simulink model "itu801_luma_chroma_fir_12bit"  (Simulink 5.0)
settings: Solver=ode45  StartTime=0.0  StopTime=60  RelTol=1e-3
libraries: simulink x4
settings Model: LastModifiedBy=thh

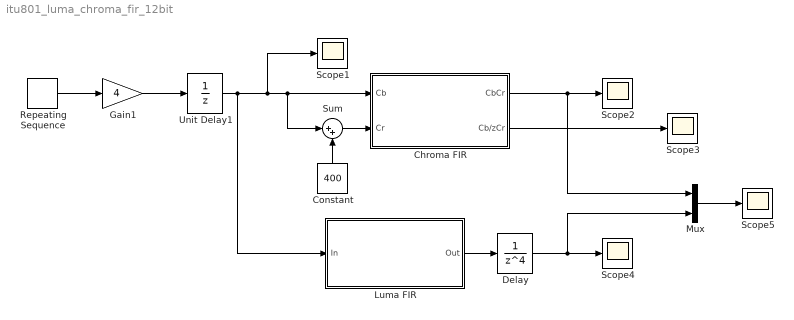
== system itu801_luma_chroma_fir_12bit ==
  Chroma FIR : Subsystem
  Constant : Constant  Orientation=up  Value=400
  Delay : DiscreteTransferFcn  Denominator=[1 0 0 0 0]
  Gain1 : Gain  Gain=4  SaturateOnIntegerOverflow=on
  Luma FIR : Subsystem
  Mux : Mux  Inputs=2
  Repeating Sequence : simulink/Sources/Repeating Sequence  rep_seq_t=[0 19 20 39 40]  rep_seq_y=[16 16 235 235 16]
  Scope{1..5} (5 alike) : Scope
      Scope1 settings: TimeRange=160  YMin=-0.2  YMax=1.2
      Scope2 settings: TimeRange=160  YMin=-1.5  YMax=4.5
      Scope3 settings: TimeRange=60  YMin=-0.2  YMax=1.2  SaveName=ScopeData3
      Scope4 settings: TimeRange=160  YMin=-0.2  YMax=1.2  SaveName=ScopeData2
      Scope5 settings: TimeRange=60  YMin=0  YMax=350  SaveName=ScopeData4
  Sum : Sum  Inputs=|++  SaturateOnIntegerOverflow=on
  Unit Delay1 : UnitDelay
  wires:
  Repeating Sequence/1 -> Gain1/1
  Sum/1 -> Chroma FIR/2(Cr)
  Constant/1 -> Sum/2
  Unit Delay1/1 -> Chroma FIR/1(Cb), Sum/1, Scope1/1, Luma FIR/1(In)
  Chroma FIR/2(Cb/zCr) -> Scope3/1
  Luma FIR/1(Out) -> Delay/1
  Mux/1 -> Scope5/1
  Gain1/1 -> Unit Delay1/1
  Delay/1 -> Scope4/1, Mux/2
  Chroma FIR/1(CbCr) -> Mux/1, Scope2/1

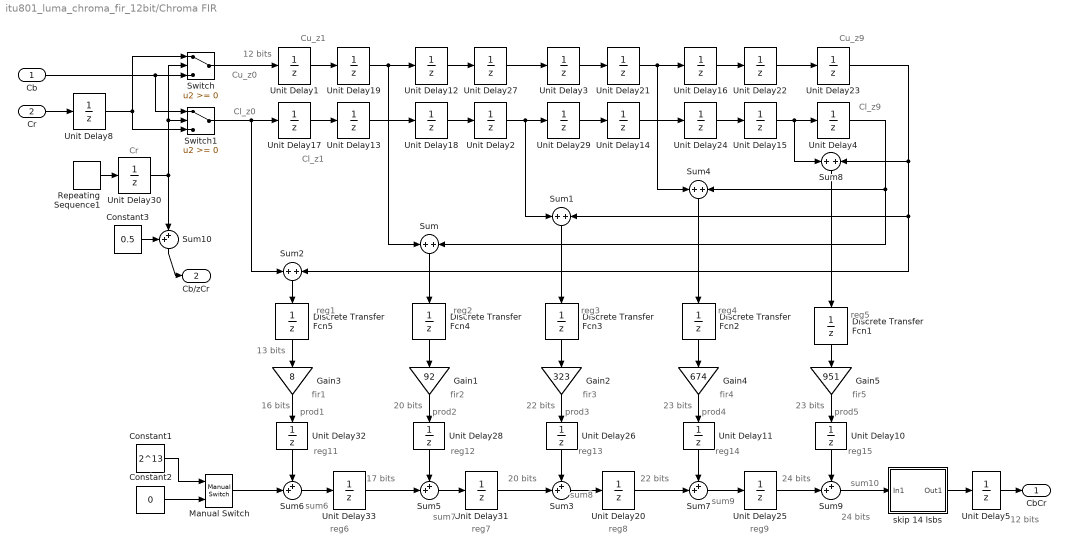
== system itu801_luma_chroma_fir_12bit/Chroma FIR ==
  note: fir1
  note: fir2
  note: fir3
  note: fir4
  note: fir5
  note: Cr
  note: 12 bits
  note: 13 bits
  note: Cu_z1
  note: Cu_z9
  note: Cl_z1
  note: Cl_z9
  note: 17 bits
  note: 20 bits
  note: 22 bits
  note: 24 bits
  note: 24 bits
  note: 12 bits
  note: reg1
  note: reg2
  note: reg3
  note: reg4
  note: reg5
  note: reg6
  note: reg7
  note: reg8
  note: reg9
  note: Cu_z0
  note: Cl_z0
  note: prod1
  note: prod2
  note: prod3
  note: prod4
  note: prod5
  note: reg11
  note: reg12
  note: reg13
  note: reg14
  note: reg15
  note: sum6
  note: sum7
  note: sum8
  note: sum9
  note: sum10
  note: 16 bits
  note: 20 bits
  note: 22 bits
  note: 23 bits
  note: 23 bits
  Cb : Inport
  Cr : Inport  Port=2
  Constant1 : Constant  Value=2^13
  Constant2 : Constant  Value=0
  Constant3 : Constant  Value=0.5
  Discrete Transfer Fcn{1..5} (5 alike) : DiscreteTransferFcn  Orientation=down  Denominator=[1 0]
  Gain1 : Gain  Orientation=down  Gain=92  SaturateOnIntegerOverflow=on
  Gain2 : Gain  Orientation=down  Gain=323  SaturateOnIntegerOverflow=on
  Gain3 : Gain  Orientation=down  Gain=8  SaturateOnIntegerOverflow=on
  Gain4 : Gain  Orientation=down  Gain=674  SaturateOnIntegerOverflow=on
  Gain5 : Gain  Orientation=down  Gain=951  SaturateOnIntegerOverflow=on
  Manual Switch : simulink/Signal Routing/Manual Switch  sw=1  action=0
  Repeating Sequence1 : simulink/Sources/Repeating Sequence  rep_seq_t=[0 1 2]  rep_seq_y=[0.5 -0.5 0.5]
  Sum{,1..2,4,8} (5 alike) : Sum  Orientation=down  SaturateOnIntegerOverflow=on
  Sum10 : Sum  Orientation=down  Inputs=++|  SaturateOnIntegerOverflow=on
  Sum{3,5..7,9} (5 alike) : Sum  Inputs=++|  SaturateOnIntegerOverflow=on
  Switch : Switch  SaturateOnIntegerOverflow=on
  Switch1 : Switch  SaturateOnIntegerOverflow=on
  Unit Delay{1..5,8,12..25,27,29,31,33} (24 alike) : UnitDelay
  Unit Delay{10..11,26,28,32} (5 alike) : UnitDelay  Orientation=down
  Unit Delay30 : UnitDelay  X0=-0.5
  skip 14 lsbs : Subsystem
  CbCr : Outport
  Cb/zCr : Outport  Port=2
  wires:
  Sum2/1 -> Discrete Transfer Fcn5/1
  Sum/1 -> Discrete Transfer Fcn4/1
  Sum1/1 -> Discrete Transfer Fcn3/1
  Gain1/1 -> Unit Delay28/1
  Gain2/1 -> Unit Delay26/1
  Unit Delay2/1 -> Unit Delay29/1, Sum1/1
  Gain3/1 -> Unit Delay32/1
  Sum6/1 -> Unit Delay33/1
  Unit Delay13/1 -> Unit Delay18/1
  Unit Delay14/1 -> Unit Delay24/1
  Discrete Transfer Fcn5/1 -> Gain3/1
  Discrete Transfer Fcn4/1 -> Gain1/1
  Discrete Transfer Fcn3/1 -> Gain2/1
  Sum5/1 -> Unit Delay31/1
  Sum4/1 -> Discrete Transfer Fcn2/1
  Gain4/1 -> Unit Delay11/1
  Discrete Transfer Fcn2/1 -> Gain4/1
  Sum3/1 -> Unit Delay20/1
  Sum8/1 -> Discrete Transfer Fcn1/1
  Gain5/1 -> Unit Delay10/1
  Discrete Transfer Fcn1/1 -> Gain5/1
  Sum7/1 -> Unit Delay25/1
  Sum9/1 -> skip 14 lsbs/1(In1)
  Unit Delay12/1 -> Unit Delay27/1
  Unit Delay18/1 -> Unit Delay2/1
  Unit Delay17/1 -> Unit Delay13/1
  Unit Delay1/1 -> Unit Delay19/1
  Unit Delay27/1 -> Unit Delay3/1
  Unit Delay3/1 -> Unit Delay21/1
  Unit Delay29/1 -> Unit Delay14/1
  Unit Delay16/1 -> Unit Delay22/1
  Unit Delay24/1 -> Unit Delay15/1
  Unit Delay22/1 -> Unit Delay23/1
  Unit Delay21/1 -> Unit Delay16/1, Sum4/1
  Unit Delay19/1 -> Unit Delay12/1, Sum/1
  Switch/1 -> Unit Delay1/1
  Switch1/1 -> Unit Delay17/1, Sum2/1
  Repeating Sequence1/1 -> Unit Delay30/1
  Cb/1 -> Switch/3, Switch1/1
  Unit Delay30/1 -> Switch/2, Switch1/2, Sum10/2
  Unit Delay23/1 -> Sum8/2, Sum2/2, Sum1/2
  Unit Delay15/1 -> Unit Delay4/1, Sum8/1
  Unit Delay25/1 -> Sum9/2
  Unit Delay20/1 -> Sum7/2
  Unit Delay31/1 -> Sum3/2
  Unit Delay33/1 -> Sum5/2
  Manual Switch/1 -> Sum6/2
  Constant1/1 -> Manual Switch/1
  Constant2/1 -> Manual Switch/2
  Cr/1 -> Unit Delay8/1
  skip 14 lsbs/1(Out1) -> Unit Delay5/1
  Unit Delay4/1 -> Sum4/2, Sum/2
  Sum10/1 -> Cb/zCr/1
  Constant3/1 -> Sum10/1
  Unit Delay5/1 -> CbCr/1
  Unit Delay8/1 -> Switch1/3, Switch/1
  Unit Delay10/1 -> Sum9/1
  Unit Delay11/1 -> Sum7/1
  Unit Delay26/1 -> Sum3/1
  Unit Delay28/1 -> Sum5/1
  Unit Delay32/1 -> Sum6/1

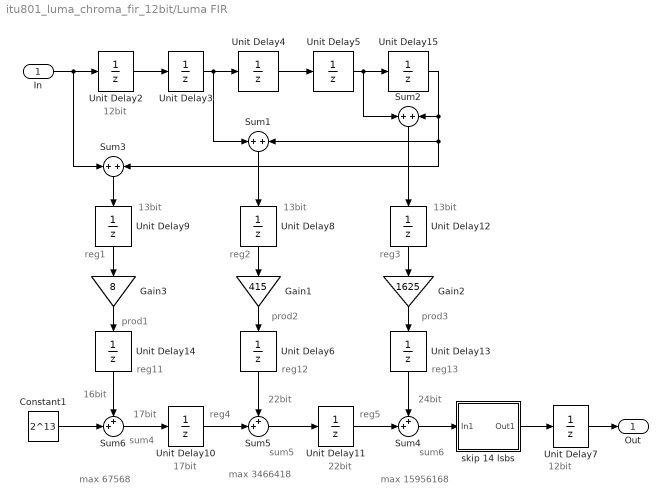
== system itu801_luma_chroma_fir_12bit/Luma FIR ==
  note: 13bit
  note: 13bit
  note: 13bit
  note: 12bit
  note: 17bit
  note: 22bit
  note: 16bit
  note: 17bit
  note: max 67568
  note: max 3466418
  note: max 15956168
  note: 22bit
  note: 24bit
  note: 12bit
  note: reg2
  note: reg1
  note: reg3
  note: reg4
  note: reg5
  note: prod1
  note: prod2
  note: prod3
  note: reg11
  note: reg12
  note: reg13
  note: sum4
  note: sum5
  note: sum6
  In : Inport
  Constant1 : Constant  Value=2^13
  Gain1 : Gain  Orientation=down  Gain=415  SaturateOnIntegerOverflow=on
  Gain2 : Gain  Orientation=down  Gain=1625  SaturateOnIntegerOverflow=on
  Gain3 : Gain  Orientation=down  Gain=8  SaturateOnIntegerOverflow=on
  Sum1 : Sum  Orientation=down  SaturateOnIntegerOverflow=on
  Sum2 : Sum  Orientation=down  SaturateOnIntegerOverflow=on
  Sum3 : Sum  Orientation=down  SaturateOnIntegerOverflow=on
  Sum4 : Sum  Inputs=++|  SaturateOnIntegerOverflow=on
  Sum5 : Sum  Inputs=++|  SaturateOnIntegerOverflow=on
  Sum6 : Sum  Inputs=++|  SaturateOnIntegerOverflow=on
  Unit Delay{2..5,7,10..11,15} (8 alike) : UnitDelay
  Unit Delay{6,8..9,12..14} (6 alike) : UnitDelay  Orientation=down
  skip 14 lsbs : Subsystem
  Out : Outport
  wires:
  Unit Delay2/1 -> Unit Delay3/1
  Unit Delay4/1 -> Unit Delay5/1
  Sum3/1 -> Unit Delay9/1
  Sum1/1 -> Unit Delay8/1
  Sum2/1 -> Unit Delay12/1
  Gain1/1 -> Unit Delay6/1
  skip 14 lsbs/1(Out1) -> Unit Delay7/1
  Sum5/1 -> Unit Delay11/1
  Sum4/1 -> skip 14 lsbs/1(In1)
  Unit Delay10/1 -> Sum5/2
  Unit Delay11/1 -> Sum4/2
  Gain2/1 -> Unit Delay13/1
  Unit Delay3/1 -> Unit Delay4/1, Sum1/1
  Gain3/1 -> Unit Delay14/1
  Sum6/1 -> Unit Delay10/1
  Constant1/1 -> Sum6/2
  Unit Delay15/1 -> Sum2/2, Sum1/2, Sum3/2
  Unit Delay5/1 -> Unit Delay15/1, Sum2/1
  Unit Delay8/1 -> Gain1/1
  Unit Delay9/1 -> Gain3/1
  Unit Delay12/1 -> Gain2/1
  In/1 -> Sum3/1, Unit Delay2/1
  Unit Delay7/1 -> Out/1
  Unit Delay13/1 -> Sum4/1
  Unit Delay6/1 -> Sum5/1
  Unit Delay14/1 -> Sum6/1

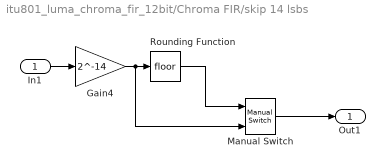
== system itu801_luma_chroma_fir_12bit/Chroma FIR/skip 14 lsbs ==
  In1 : Inport
  Gain4 : Gain  Gain=2^-14  SaturateOnIntegerOverflow=on
  Manual Switch : simulink/Signal Routing/Manual Switch  sw=1  action=0
  Rounding Function : Rounding
  Out1 : Outport
  wires:
  Gain4/1 -> Rounding Function/1, Manual Switch/2
  In1/1 -> Gain4/1
  Manual Switch/1 -> Out1/1
  Rounding Function/1 -> Manual Switch/1

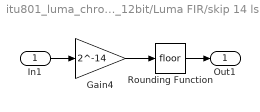
== system itu801_luma_chroma_fir_12bit/Luma FIR/skip 14 lsbs ==
  In1 : Inport
  Gain4 : Gain  Gain=2^-14  SaturateOnIntegerOverflow=on
  Rounding Function : Rounding
  Out1 : Outport
  wires:
  Gain4/1 -> Rounding Function/1
  In1/1 -> Gain4/1
  Rounding Function/1 -> Out1/1
